simulink model "spsim"  (R2013a)
settings: Solver=ode45  StartTime=0.0  StopTime=Tf  RelTol=1e-3
values from neighbouring files (symbols this model uses):
  b = 0.001    [ta1.m]    (also in ta3.m = 0.1)
  g = 9.8    [ta1.m]    (also in ta3.m)
  l = 0.5    [ta1.m]    (also in ta3.m)
  m = 0.1    [ta1.m]    (also in ta3.m)
settings Model: Creator=Al_Farabi  LastModifiedBy=Al_Farabi

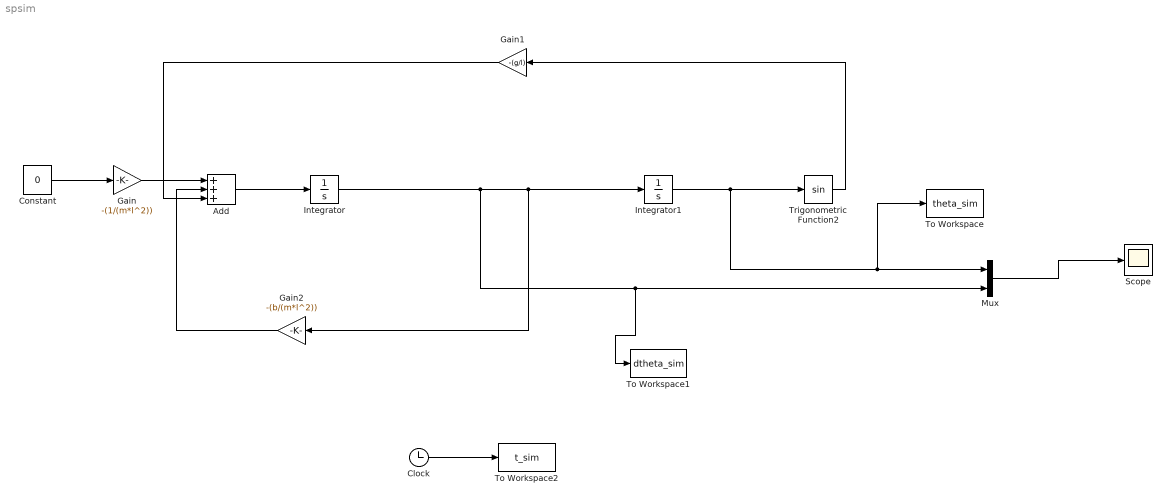
== system spsim ==
  Add : Sum  Inputs=+++
  Clock : Clock
  Constant : Constant  Value=0
  Gain : Gain  Gain=-(1/(m*l^2))
  Gain1 : Gain  Gain=-(g/l)
  Gain2 : Gain  Gain=-(b/(m*l^2))
  Integrator : Integrator
  Integrator1 : Integrator
  Mux : Mux  Inputs=2
  Scope : Scope
  To Workspace : ToWorkspace  VariableName=theta_sim  SampleTime=-1
  To Workspace1 : ToWorkspace  VariableName=dtheta_sim  SampleTime=-1
  To Workspace2 : ToWorkspace  VariableName=t_sim  SampleTime=-1
  Trigonometric Function2 : Trigonometry
  wires:
  Add/1 -> Integrator/1
  Integrator/1 -> To Workspace1/1, Mux/2, Gain2/1, Integrator1/1
  Constant/1 -> Gain/1
  Gain/1 -> Add/1
  Gain2/1 -> Add/2
  Gain1/1 -> Add/3
  Integrator1/1 -> Mux/1, To Workspace/1, Trigonometric Function2/1
  Trigonometric Function2/1 -> Gain1/1
  Mux/1 -> Scope/1
  Clock/1 -> To Workspace2/1
